simulink model "SMC_POS_SMC_Att"  (R2024b)
settings: Solver=FixedStepDiscrete  StartTime=0.0  StopTime=45  FixedStep=1/250  RelTol=1e-3
values from neighbouring files (symbols this model uses):
  a1 = 3.5524    [Parameter_SMC.m]
  a2 = 10.000    (= 10)    [Parameter_SMC.m]
  a3 = 8.1910    (= 8.191)    [Parameter_SMC.m]
  a4 = 2.7640    (= 2.764)    [Parameter_SMC.m]
  b3 = 0.6373    [Parameter_SMC.m]
  b4 = 0.0223    [Parameter_SMC.m]
  b_1x = 0.7426    [Parameter_SMC.m]
  b_1y = 0.5930    (= 0.593)    [Parameter_SMC.m]
  b_2x = 1.4305    [Parameter_SMC.m]
  b_2y = 1.0895    [Parameter_SMC.m]
  c_x = 0.2871    [Parameter_SMC.m]
  c_y = 0.3867    [Parameter_SMC.m]
  epsilon_1_a = 0.5    [Parameter_SMC.m]
  epsilon_1_b = 0.5    [Parameter_SMC.m]
  epsilon_2 = 0.5    [Parameter_SMC.m]
  epsilon_2_b = 0.5    [Parameter_SMC.m]
  g = 9.81    [Parameter_SMC.m]
  Jx = 0.005    [Parameter_SMC.m]
  Jy = 0.005    [Parameter_SMC.m]
  Jz = 0.009    [Parameter_SMC.m]
  K1 = 0.01    [Parameter_SMC.m]
  k1 = 0.001    [Parameter_SMC.m]
  K2 = 0    [Parameter_SMC.m]
  k2 = a1    (= 3.5524)    [Parameter_SMC.m]
  k3 = 0.1    [Parameter_SMC.m]
  k4 = 0.5000    (= 0.5)    [Parameter_SMC.m]
  k5 = 0.0388    [Parameter_SMC.m]
  k6 = Jx * a3 / (l * sqrt(8) * Tmax)    [Parameter_SMC.m]
  k7 = 0.3147    [Parameter_SMC.m]
  k8 = a4 * Jz / (4 * Qmax)    (= 0.12438)    [Parameter_SMC.m]
  k_ob = 1    [Parameter_SMC.m]
  l = 0.33/2    (= 0.165)    [Parameter_SMC.m]
  m = 0.8    [Parameter_SMC.m]
  PWM_max = 2000    [Parameter_SMC.m]
  PWM_min = 1000    [Parameter_SMC.m]
  Qmax = 0.05    [Parameter_SMC.m]
  Tmax = 4    [Parameter_SMC.m]
undefined symbols (not defined in the file or in its folder): d_1_x, DiscIntNeverNeededParam, k_1_a, k_1_b, k_2_a, k_2_b, K_4, Q_max, T_max
libraries: simulink x13, slpidlib x3
(part 2 of 2)

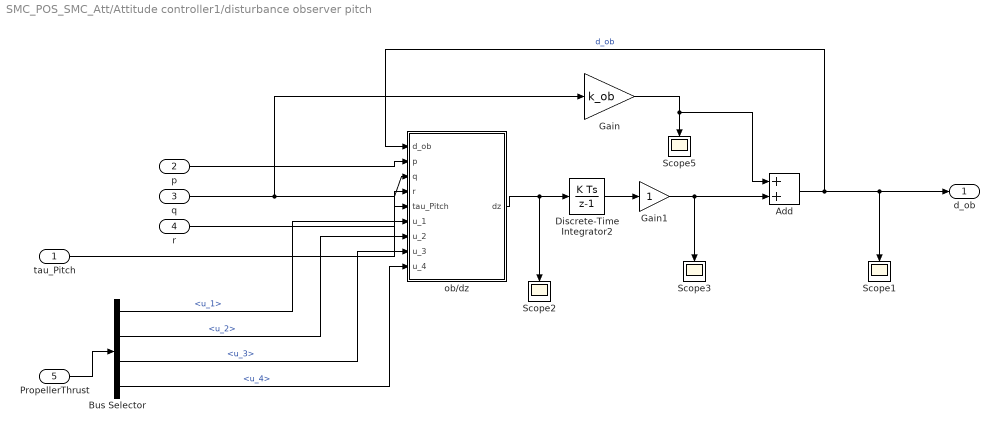
== system SMC_POS_SMC_Att/Attitude controller1/disturbance observer pitch ==
  tau_Pitch : Inport
  "p " : Inport  Port=2
  q : Inport  Port=3
  r : Inport  Port=4
  PropellerThrust : Inport  Port=5
  Add : Sum
  Bus Selector : BusSelector  OutputSignals=u_1,u_2,u_3,u_4
  Discrete-Time Integrator2 : DiscreteIntegrator  SampleTime=-1  ICPrevOutput=DiscIntNeverNeededParam  ICPrevScaledInput=DiscIntNeverNeededParam
  Gain : Gain  Gain=k_ob
  Gain1 : Gain
  Scope{1..3,5} (4 alike) : Scope
  ob/dz : MATLAB Function  TreatAsAtomicUnit=on
  d_ob : Outport
  wires:
  ob/dz/1(dz) -> Discrete-Time Integrator2/1, Scope2/1
  Discrete-Time Integrator2/1 -> Gain1/1
  Gain/1 -> Scope5/1, Add/1
  Add/1 -> Scope1/1, d_ob/1, ob/dz/1(d_ob)  "d_ob"
  Gain1/1 -> Add/2, Scope3/1
  tau_Pitch/1 -> ob/dz/5(tau_Pitch)
  r/1 -> ob/dz/4(r)
  q/1 -> ob/dz/3(q), Gain/1
  "p "/1 -> ob/dz/2(p)
  PropellerThrust/1 -> Bus Selector/1
  Bus Selector/1 -> ob/dz/6(u_1)  "<u_1>"
  Bus Selector/2 -> ob/dz/7(u_2)  "<u_2>"
  Bus Selector/3 -> ob/dz/8(u_3)  "<u_3>"
  Bus Selector/4 -> ob/dz/9(u_4)  "<u_4>"

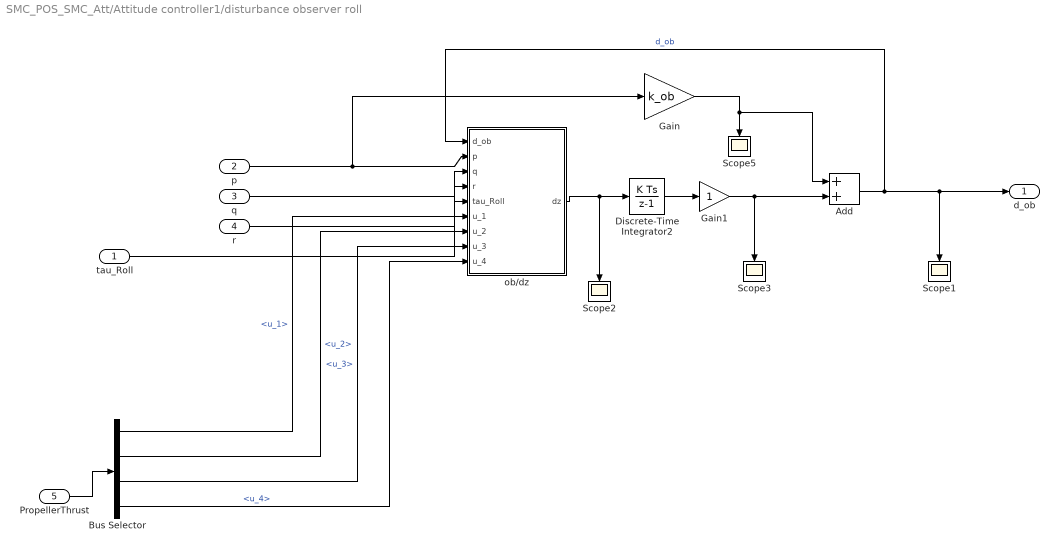
== system SMC_POS_SMC_Att/Attitude controller1/disturbance observer roll ==
  tau_Roll : Inport
  "p " : Inport  Port=2
  q : Inport  Port=3
  r : Inport  Port=4
  PropellerThrust : Inport  Port=5
  Add : Sum
  Bus Selector : BusSelector  OutputSignals=u_1,u_2,u_3,u_4
  Discrete-Time Integrator2 : DiscreteIntegrator  SampleTime=-1  ICPrevOutput=DiscIntNeverNeededParam  ICPrevScaledInput=DiscIntNeverNeededParam
  Gain : Gain  Gain=k_ob
  Gain1 : Gain
  Scope{1..3,5} (4 alike) : Scope
  ob/dz : MATLAB Function  TreatAsAtomicUnit=on
  d_ob : Outport
  wires:
  ob/dz/1(dz) -> Discrete-Time Integrator2/1, Scope2/1
  Discrete-Time Integrator2/1 -> Gain1/1
  Gain/1 -> Scope5/1, Add/1
  Add/1 -> Scope1/1, d_ob/1, ob/dz/1(d_ob)  "d_ob"
  Gain1/1 -> Add/2, Scope3/1
  tau_Roll/1 -> ob/dz/5(tau_Roll)
  r/1 -> ob/dz/4(r)
  q/1 -> ob/dz/3(q)
  "p "/1 -> Gain/1, ob/dz/2(p)
  Bus Selector/4 -> ob/dz/9(u_4)  "<u_4>"
  Bus Selector/3 -> ob/dz/8(u_3)  "<u_3>"
  Bus Selector/1 -> ob/dz/6(u_1)  "<u_1>"
  PropellerThrust/1 -> Bus Selector/1
  Bus Selector/2 -> ob/dz/7(u_2)  "<u_2>"

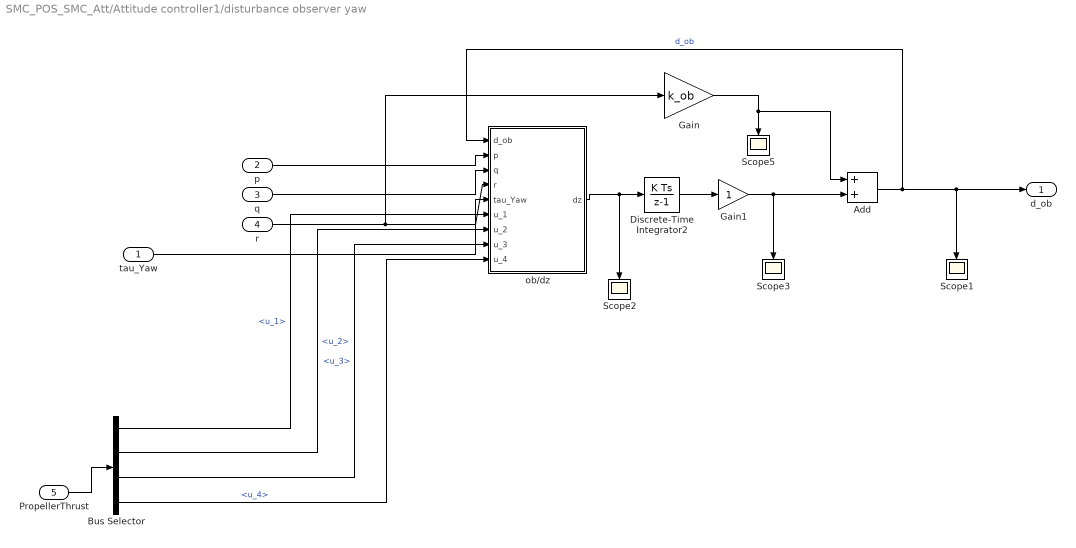
== system SMC_POS_SMC_Att/Attitude controller1/disturbance observer yaw ==
  tau_Yaw : Inport
  "p " : Inport  Port=2
  q : Inport  Port=3
  r : Inport  Port=4
  PropellerThrust : Inport  Port=5
  Add : Sum
  Bus Selector : BusSelector  OutputSignals=u_1,u_2,u_3,u_4
  Discrete-Time Integrator2 : DiscreteIntegrator  SampleTime=-1  ICPrevOutput=DiscIntNeverNeededParam  ICPrevScaledInput=DiscIntNeverNeededParam
  Gain : Gain  Gain=k_ob
  Gain1 : Gain
  Scope{1..3,5} (4 alike) : Scope
  ob/dz : MATLAB Function  TreatAsAtomicUnit=on
  d_ob : Outport
  wires:
  ob/dz/1(dz) -> Discrete-Time Integrator2/1, Scope2/1
  Discrete-Time Integrator2/1 -> Gain1/1
  Gain/1 -> Scope5/1, Add/1
  Add/1 -> Scope1/1, d_ob/1, ob/dz/1(d_ob)  "d_ob"
  Gain1/1 -> Add/2, Scope3/1
  tau_Yaw/1 -> ob/dz/5(tau_Yaw)
  r/1 -> Gain/1, ob/dz/4(r)
  q/1 -> ob/dz/3(q)
  "p "/1 -> ob/dz/2(p)
  Bus Selector/4 -> ob/dz/9(u_4)  "<u_4>"
  Bus Selector/3 -> ob/dz/8(u_3)  "<u_3>"
  Bus Selector/1 -> ob/dz/6(u_1)  "<u_1>"
  PropellerThrust/1 -> Bus Selector/1
  Bus Selector/2 -> ob/dz/7(u_2)  "<u_2>"

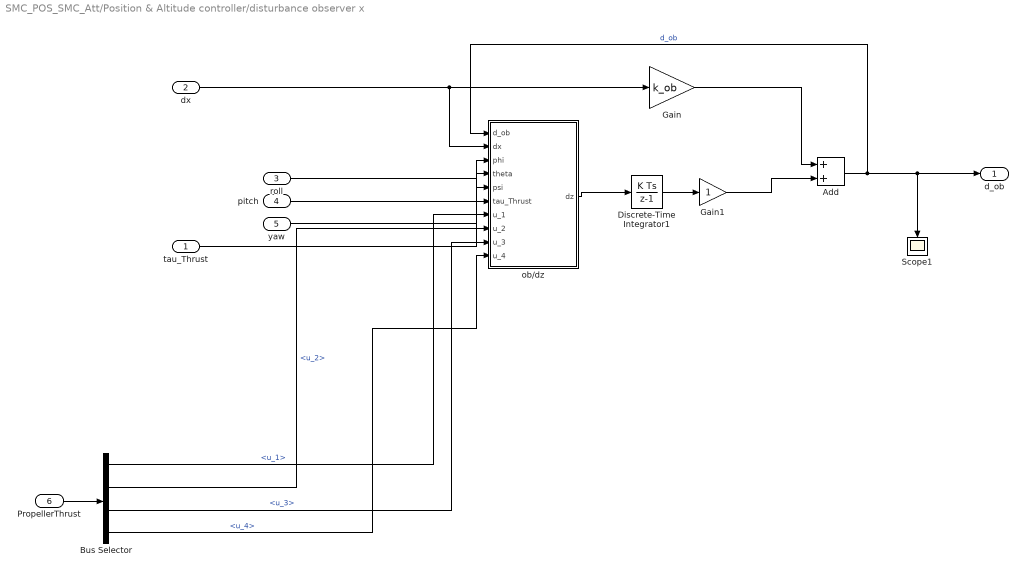
== system SMC_POS_SMC_Att/Position & Altitude controller/disturbance observer x ==
  tau_Thrust : Inport
  dx : Inport  Port=2
  "roll " : Inport  Port=3
  pitch : Inport  Port=4
  yaw : Inport  Port=5
  PropellerThrust : Inport  Port=6
  Add : Sum
  Bus Selector : BusSelector  OutputSignals=u_1,u_2,u_3,u_4
  Discrete-Time Integrator1 : DiscreteIntegrator  SampleTime=-1  ICPrevOutput=DiscIntNeverNeededParam  ICPrevScaledInput=DiscIntNeverNeededParam
  Gain : Gain  Gain=k_ob
  Gain1 : Gain
  Scope1 : Scope
  ob/dz : MATLAB Function  TreatAsAtomicUnit=on
  d_ob : Outport
  wires:
  tau_Thrust/1 -> ob/dz/6(tau_Thrust)
  ob/dz/1(dz) -> Discrete-Time Integrator1/1
  Discrete-Time Integrator1/1 -> Gain1/1
  Gain/1 -> Add/1
  Add/1 -> Scope1/1, d_ob/1, ob/dz/1(d_ob)  "d_ob"
  Gain1/1 -> Add/2
  "roll "/1 -> ob/dz/3(phi)
  pitch/1 -> ob/dz/4(theta)
  yaw/1 -> ob/dz/5(psi)
  dx/1 -> ob/dz/2(dx), Gain/1
  Bus Selector/2 -> ob/dz/8(u_2)  "<u_2>"
  PropellerThrust/1 -> Bus Selector/1
  Bus Selector/4 -> ob/dz/10(u_4)  "<u_4>"
  Bus Selector/1 -> ob/dz/7(u_1)  "<u_1>"
  Bus Selector/3 -> ob/dz/9(u_3)  "<u_3>"

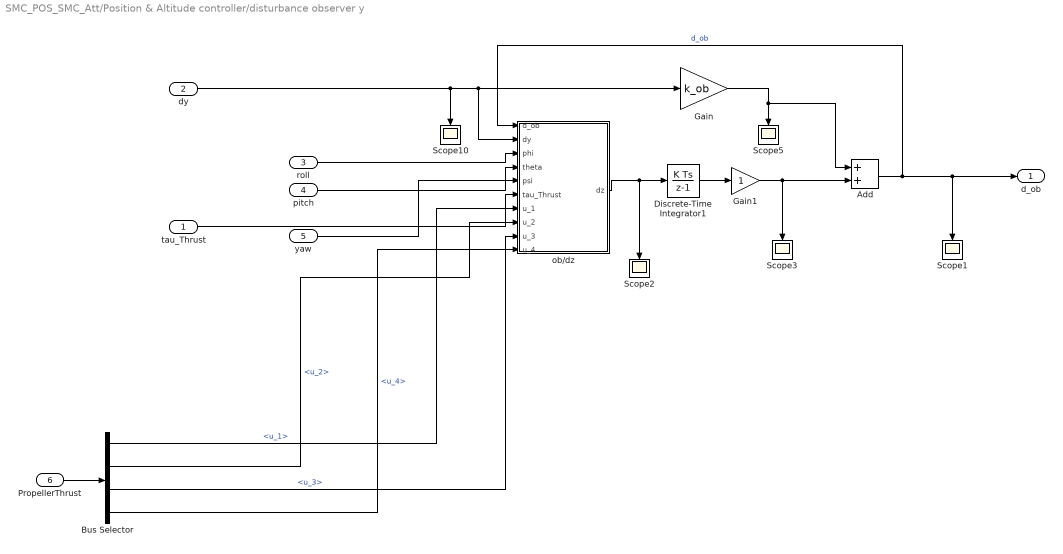
== system SMC_POS_SMC_Att/Position & Altitude controller/disturbance observer y ==
  tau_Thrust : Inport
  dy : Inport  Port=2
  "roll " : Inport  Port=3
  pitch : Inport  Port=4
  yaw : Inport  Port=5
  PropellerThrust : Inport  Port=6
  Add : Sum
  Bus Selector : BusSelector  OutputSignals=u_1,u_2,u_3,u_4
  Discrete-Time Integrator1 : DiscreteIntegrator  SampleTime=-1  ICPrevOutput=DiscIntNeverNeededParam  ICPrevScaledInput=DiscIntNeverNeededParam
  Gain : Gain  Gain=k_ob
  Gain1 : Gain
  Scope{1..3,5,10} (5 alike) : Scope
  ob/dz : MATLAB Function  TreatAsAtomicUnit=on
  d_ob : Outport
  wires:
  tau_Thrust/1 -> ob/dz/6(tau_Thrust)
  ob/dz/1(dz) -> Discrete-Time Integrator1/1, Scope2/1
  Gain/1 -> Scope5/1, Add/1
  Add/1 -> Scope1/1, d_ob/1, ob/dz/1(d_ob)  "d_ob"
  Gain1/1 -> Add/2, Scope3/1
  "roll "/1 -> ob/dz/3(phi)
  pitch/1 -> ob/dz/4(theta)
  yaw/1 -> ob/dz/5(psi)
  dy/1 -> ob/dz/2(dy), Gain/1, Scope10/1
  Discrete-Time Integrator1/1 -> Gain1/1
  Bus Selector/2 -> ob/dz/8(u_2)  "<u_2>"
  PropellerThrust/1 -> Bus Selector/1
  Bus Selector/4 -> ob/dz/10(u_4)  "<u_4>"
  Bus Selector/1 -> ob/dz/7(u_1)  "<u_1>"
  Bus Selector/3 -> ob/dz/9(u_3)  "<u_3>"

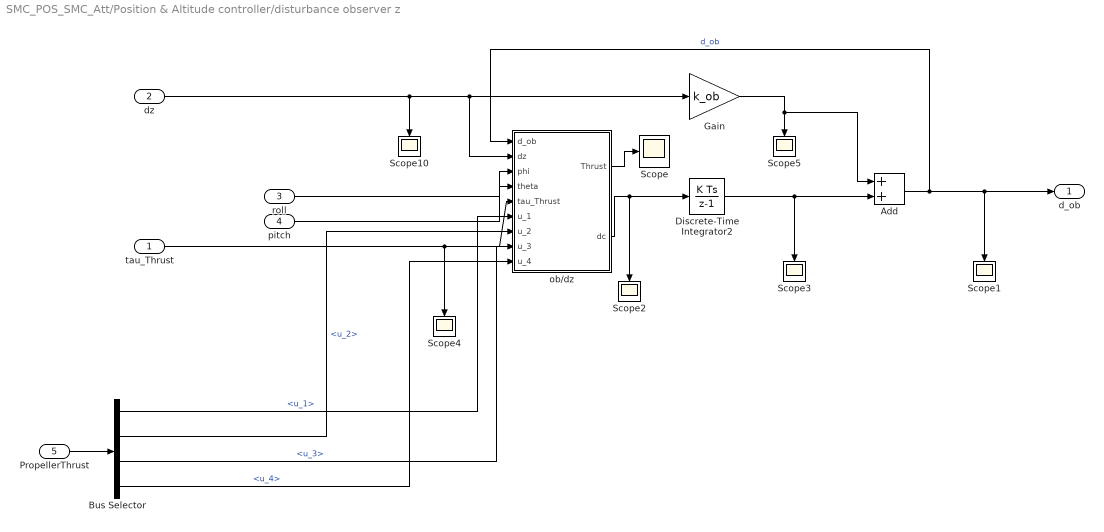
== system SMC_POS_SMC_Att/Position & Altitude controller/disturbance observer z ==
  tau_Thrust : Inport
  dz : Inport  Port=2
  "roll " : Inport  Port=3
  pitch : Inport  Port=4
  PropellerThrust : Inport  Port=5
  Add : Sum
  Bus Selector : BusSelector  OutputSignals=u_1,u_2,u_3,u_4
  Discrete-Time Integrator2 : DiscreteIntegrator  SampleTime=-1  ICPrevOutput=DiscIntNeverNeededParam  ICPrevScaledInput=DiscIntNeverNeededParam
  Gain : Gain  Gain=k_ob
  Scope{,1..5,10} (7 alike) : Scope
  ob/dz : MATLAB Function  TreatAsAtomicUnit=on
  d_ob : Outport
  wires:
  Gain/1 -> Scope5/1, Add/1
  Add/1 -> Scope1/1, d_ob/1, ob/dz/1(d_ob)  "d_ob"
  "roll "/1 -> ob/dz/3(phi)
  pitch/1 -> ob/dz/4(theta)
  tau_Thrust/1 -> Scope4/1, ob/dz/5(tau_Thrust)
  dz/1 -> Gain/1, ob/dz/2(dz), Scope10/1
  ob/dz/2(dc) -> Discrete-Time Integrator2/1, Scope2/1
  Discrete-Time Integrator2/1 -> Add/2, Scope3/1
  ob/dz/1(Thrust) -> Scope/1
  Bus Selector/4 -> ob/dz/9(u_4)  "<u_4>"
  Bus Selector/3 -> ob/dz/8(u_3)  "<u_3>"
  Bus Selector/1 -> ob/dz/6(u_1)  "<u_1>"
  PropellerThrust/1 -> Bus Selector/1
  Bus Selector/2 -> ob/dz/7(u_2)  "<u_2>"

== matlab function SMC_POS_SMC_Att/Position & Altitude controller/Calculate roll and pitch angles  ==
  data: u1 input; theta output; u2 input; psi input; phi output
function [theta,phi] = fcn(u1,u2,psi)
int1=u1*sin(psi)-u2*cos(psi);
if int1 >1 
    int1 =1; 
else if int1 <-1 
        int1=-1;
    else 
        int1=int1;
    end
end
phi=asin(int1);
if phi>1.5 
    phi_2=1.5;
else if phi<-1.5
        phi_2=-1.5;
    else
        phi_2=phi;
    end
end
int2=(u1*cos(psi)+u2*sin(psi))/cos(phi_2);
if int2 >1 
    int2 =1; 
else if int2 <-1 
        int2=-1;
    else 
        int2=int2;
    end
end
theta=asin(int2);
end

== matlab function SMC_POS_SMC_Att/Attitude controller1/MATLAB Function6 ==
  data: roll input; p output; pitch input; yaw input; q output; r output; droll input; dpitch input; dyaw input
function [p, q, r] = fcn(roll,pitch,yaw, droll, dpitch, dyaw)
p=droll-sin(pitch)*dyaw;
q=cos(roll)*dpitch+cos(pitch)*sin(roll)*dyaw;
r=-sin(roll)*dpitch+cos(pitch)*cos(roll)*dyaw;
end

== matlab function SMC_POS_SMC_Att/Position & Altitude controller/Sliding Mode Surface2 ==
  data: error_dz output; sz output; error_z input; dz input; a2 parameter; epsilon_2_b parameter; des_dz input
function [error_dz,sz] = fcn(error_z,dz, a2, epsilon_2_b,des_dz)
error_dz=dz-des_dz;

sz=(a2*error_z+error_dz)/epsilon_2_b;

end

== matlab function SMC_POS_SMC_Att/Position & Altitude controller/Control law3 ==
  data: error_dz input; K1 parameter; k3 parameter; k4 parameter; sgn input; s input; dz input; u output; g parameter; m parameter; phi input; theta input; Tmax parameter; error_z input; b3 parameter; b4 parameter; des_ddz input
 function u  = fcn( error_dz,K1, k3,k4,sgn,s,dz,g, m, phi, theta,Tmax,error_z, b3, b4, des_ddz)
 
 kint=(b3*abs(error_z)+b4*abs(error_dz));
 
 if kint<k3
    kint=k3;
end
if abs(s)<1
u=kint*s+k4/(cos(theta)*cos(phi))*(error_dz)+(-K1*dz*abs(dz)+m*g-m*des_ddz)/(4*Tmax*cos(phi)*cos(theta))+1;
else
%   u=k_3_b*sgn+k_4_b*(error_dz)+(K_3*dz+m*g)/(4*T_max*cos(phi)*cos(theta))+1
    u=kint*sgn+k4/(cos(theta)*cos(phi))*(error_dz)+(-K1*dz*abs(dz)+m*g-m*des_ddz)/(4*Tmax*cos(phi)*cos(theta))+1;
end

== matlab function SMC_POS_SMC_Att/Position & Altitude controller/Sliding Mode Surface ==
  data: sx output; error_x input; error_dx output; error_y input; dx input; dy input; error_dy output; sy output; a1 parameter; epsilon_2 parameter; des_dx input; des_dy input
function [sx,error_dx,error_dy,sy] = fcn(error_x,error_y,dx,dy,a1,epsilon_2,des_dx, des_dy)
error_dx=dx-des_dx;
error_dy=dy-des_dy;
sx=(a1*error_x+error_dx)/epsilon_2;
sy=(a1*error_y+error_dy)/epsilon_2;

end

== matlab function SMC_POS_SMC_Att/Attitude controller1/MATLAB Function ==
  data: error_phi input; dphi input; dtheta input; s_phi output; error_theta input; error_dphi output; s_theta output; error_dtheta output; epsilon_1_a parameter; a3 parameter; des_dphi input; des_dtheta input
function [s_phi,error_dphi,s_theta,error_dtheta] = fcn(error_phi, dphi, dtheta,error_theta,epsilon_1_a, a3, des_dphi, des_dtheta)
error_dphi=dphi-des_dphi;
error_dtheta=dtheta-des_dtheta;

s_phi=(a3*error_phi+error_dphi)/epsilon_1_a;
s_theta=(a3*error_theta+error_dtheta)/epsilon_1_a;

== matlab function SMC_POS_SMC_Att/Attitude controller1/derivative1/MATLAB Function7 ==
  data: u input; y output
function y = fcn(u)
if abs(u)>30 
    u=0;
end
y = u;

== matlab function SMC_POS_SMC_Att/Position & Altitude controller/Control law1 ==
  data: error_x input; d_ob input; dx input; K1 parameter; k1 parameter; k2 parameter; sgn input; s input; error_dx input; g parameter; m parameter; u output; theta input; phi input; b_1x parameter; b_2x parameter; des_ddx input; c_x parameter
 function u = fcn(error_x, d_ob,dx,K1, k1,k2,sgn,s,error_dx,g, m, theta, phi, b_1x, b_2x, des_ddx, c_x)

%      if abs(s)<1
%  u=(k_3*s+k_4*(error_dx)+K_1*dx/(m*g))-d_ob*m*reci_Thrust
% else
%      u=(k_3*sgn+k_4*(error_dx)+K_1*dx/(m*g))-d_ob*m*reci_Thrust
% 
%      end
% (k_3-0.2*(1.5^(-abs(error_x))-1))
%      if abs(s)<1
%  u=(k_3*s+k_4*(error_dx)+K_1*dx/(m*g))-d_ob*m*reci_Thrust
% else
%      u=((k_3-0.2*(1.5^(-abs(error_x))-1))*sgn+k_4*(error_dx)+K_1*dx/(m*g))-d_ob*m*reci_Thrust
% 
%      end
% %   kint=(0.08*abs(error_x)-0.13*abs(error_dx));clear all


  kint=(b_1x*abs(error_x)+b_2x*abs(error_dx));

if kint<k1
    kint=k1;
end
if abs(s)<1
 u=(kint*(cos(phi)*cos(theta)/g)*s+k2*(cos(phi)*cos(theta)/g)*error_dx-K1*(cos(phi)*cos(theta)/(m*g))*dx*abs(dx)-(cos(phi)*cos(theta)/g)*des_ddx+c_x*(cos(phi)*cos(theta)/g)*s)+d_ob*(cos(phi)*cos(theta)/g);
%   u=(kint*s+k_4*cos(theta)*cos(phi)*error_dx+K_1*cos(theta)*cos(phi)*dx/(m*g)-cos(theta)*cos(phi)*des_ddx/g)-d_ob*m*reci_Thrust
else    
% u=((k_3-0.2*(1.5^(-abs(error_x))-1))*sgn+k_4*(error_dx)+K_1*dx/(m*g))-d_ob*m*reci_Thrust
% u=((0.05*abs(error_x)-0.065*abs(error_dx))*sgn+k_4*(error_dx)+K_1*dx/(m*g))-d_ob*m*reci_Thrust
 u=(kint*(cos(phi)*cos(theta)/g)*sgn+k2*(cos(phi)*cos(theta)/g)*error_dx-K1*(cos(phi)*cos(theta)/(m*g))*dx*abs(dx)-(cos(phi)*cos(theta)/g)*des_ddx+c_x*(cos(phi)*cos(theta)/g)*s)+d_ob*(cos(phi)*cos(theta)/g);
%   u=(kint*sgn+k_4*cos(theta)*cos(phi)*error_dx+K_1*cos(theta)*cos(phi)*dx/(m*g)-cos(theta)*cos(phi)*des_ddx/g)-d_ob*m*reci_Thrust
end

== matlab function SMC_POS_SMC_Att/Attitude controller1/derivative3/MATLAB Function7 ==
  data: u input; y output
function y = fcn(u)
if abs(u)>30 
    u=0;
end
y = u;

== matlab function SMC_POS_SMC_Att/Attitude controller1/MATLAB Function3 ==
  data: error input; s_psi output; dpsi input; error_dpsi output; a4 parameter; epsilon_1_b parameter; des_dpsi input
function [s_psi,error_dpsi] = fcn(error,dpsi,a4, epsilon_1_b, des_dpsi)
error_psi=error;
error_dpsi=dpsi-des_dpsi;
s_psi=(a4*error_psi+error_dpsi)/epsilon_1_b;

== matlab function SMC_POS_SMC_Att/Attitude controller1/derivative10/MATLAB Function7 ==
  data: u input; y output
function y = fcn(u)
if abs(u)>30 
    u=0;
end
y = u;

== matlab function SMC_POS_SMC_Att/Position & Altitude controller/disturbance observer x/ob//dz ==
  data: d_ob input; dx input; m parameter; PWM_min parameter; PWM_max parameter; phi input; theta input; psi input; dz output; Tmax parameter; tau_Thrust input; k_ob parameter; K1 parameter; u_1 input; u_2 input; u_3 input; u_4 input
 function  dz = fcn(d_ob, dx, m, PWM_min, PWM_max, phi,theta,psi, Tmax, tau_Thrust, k_ob, K1, u_1, u_2, u_3, u_4)
u_x=sin(phi)*sin(psi)+cos(phi)*sin(theta)*cos(psi);
Thrust = -Tmax*(4000*(tau_Thrust)-4*PWM_min)/(PWM_max-PWM_min);
% dz = -k_ob*d_ob - k_ob*(1/m*u_x*Thrust- (K_1*dx)/m);
% test= k_ob*1/m*u_x*Thrust;
dz = -k_ob*d_ob - k_ob*(1/m*u_x*(-Tmax*(u_1+u_2+u_3+u_4))- (K1*dx*abs(dx))/m);

end

== matlab function SMC_POS_SMC_Att/Position & Altitude controller/disturbance observer y/ob//dz ==
  data: d_ob input; dy input; m parameter; PWM_min parameter; PWM_max parameter; phi input; theta input; psi input; dz output; Tmax parameter; tau_Thrust input; k_ob parameter; K1 parameter; u_1 input; u_2 input; u_3 input; u_4 input
 function dz  = fcn(d_ob, dy, m, PWM_min, PWM_max, phi,theta,psi, Tmax, tau_Thrust, k_ob, K1, u_1, u_2, u_3, u_4)
u_y=-sin(phi)*cos(psi)+cos(phi)*sin(theta)*sin(psi);
Thrust = -Tmax*(4000*(tau_Thrust)-4*PWM_min)/(PWM_max-PWM_min);
% dz = -k_ob*d_ob - k_ob*(1/m*u_y*Thrust- (K_1*dy)/m);
% test= k_ob*1/m*u_x*Thrust;
dz = -k_ob*d_ob - k_ob*(1/m*u_y*(-Tmax*(u_1+u_2+u_3+u_4))- (K1*dy*abs(dy))/m);

end

== matlab function SMC_POS_SMC_Att/Attitude controller1/disturbance observer pitch/ob//dz ==
  data: d_ob input; Tmax parameter; k_ob parameter; K2 parameter; p input; dz output; q input; r input; tau_Pitch input; Jz parameter; Jy parameter; Jx parameter; l parameter; u_1 input; u_2 input; u_3 input; u_4 input
 function dz  = fcn(d_ob,  Tmax,  k_ob, K2, p, q, r, tau_Pitch, Jz, Jy, Jx, l, u_1, u_2, u_3, u_4)

%dz = -k_ob*d_ob - k_ob/Jy*(-T_max*l*sqrt(2)/2*(4*tau_Pitch)-K_2*q-p*r*(Jx-Jz));

dz = -k_ob*d_ob - k_ob/Jy*(-Tmax*(u_2*(l*sqrt(2)/2)+ u_4*(l*sqrt(2)/2)- u_1*(l*sqrt(2)/2)- u_3*(l*sqrt(2)/2))-K2*q*abs(q)-p*r*(Jx-Jz));

end

== matlab function SMC_POS_SMC_Att/Dynamic model /Dynamic model ==
  data: channel input double size=4; ddx output size=1; phi input; theta input; psi input; Qmax parameter; Tmax parameter; g parameter; dx input; dy input; dz input; p input; q input; r input; Jy parameter; Jz parameter; Jx parameter; m parameter; ddy output size=1; ddz output size=1; dp output size=1; dq output size=1; dr output size=1; K1 parameter; K2 parameter; l parameter; PWM_max parameter; PWM_min parameter; d_f_x input; d_f_y input; d_f_z input; d_t_p input; d_t_q input; d_t_r input; bias_x input; bias_y input; u_1 output size=1; u_2 output size=1; u_3 output size=1; u_4 output size=1
 function [ddx,ddy,ddz,dp,dq,dr,u_1,u_2,u_3,u_4] =...
     fcn(channel,phi,theta,psi,Qmax,Tmax,g,dx,dy,dz,p,q,r, Jy, Jz, Jx, m,K1, K2, l, PWM_max, PWM_min, d_f_x, d_f_y, d_f_z, d_t_p, d_t_q, d_t_r, bias_x, bias_y)
 
%propeller speed, dutycycle
for index = 1:4
    if channel(index)<PWM_min
    channel(index)=PWM_min;
            else if channel(index)>PWM_max
             channel(index)=PWM_max;
                else
             channel(index)=channel(index);
                 end
    end
end
%,u_2,u_3,u_4
u_1=(channel(1)-PWM_min)/(PWM_max-PWM_min);
u_2=(channel(2)-PWM_min)/(PWM_max-PWM_min);
u_3=(channel(3)-PWM_min)/(PWM_max-PWM_min);
u_4=(channel(4)-PWM_min)/(PWM_max-PWM_min);

ddx = (sin(phi)*sin(psi)+cos(phi)*sin(theta)*cos(psi))*(-Tmax*(u_1+u_2+u_3+u_4))/m - (K1*dx*abs(dx))/m + d_f_x;
ddy = (-sin(phi)*cos(psi)+cos(phi)*sin(theta)*sin(psi))*(-Tmax*(u_1+u_2+u_3+u_4))/m - (K1*dy*abs(dy))/m + d_f_y;
ddz = g + (cos(phi)*cos(theta))*(-Tmax*(u_1+u_2+u_3+u_4))/m - (K1*dz*abs(dz))/m + d_f_z;

% roll
dp = (-Tmax*(u_1*(l*sqrt(2)/2-bias_y)+ u_4*(l*sqrt(2)/2-bias_y)- u_2*(l*sqrt(2)/2+bias_y)- u_3*(l*sqrt(2)/2+bias_y)) - K2*p*abs(p) - q*r*(Jz-Jy))/Jx + d_t_p;

% pitch
dq = (-Tmax*(u_2*(l*sqrt(2)/2+bias_x)+ u_4*(l*sqrt(2)/2+bias_x)- u_1*(l*sqrt(2)/2-bias_x)- u_3*(l*sqrt(2)/2-bias_x)) - K2*q*abs(q) - p*r*(Jx-Jz))/Jy + d_t_q;

%yaw
dr = (Qmax*(u_1+u_2-u_3-u_4) - K2*r*abs(r) - p*q*(Jy-Jx))/Jz + d_t_r;

== matlab function SMC_POS_SMC_Att/Position & Altitude controller/disturbance observer z/ob//dz ==
  data: Thrust output; d_ob input; dz input; m parameter; PWM_min parameter; PWM_max parameter; phi input; theta input; dc output; Tmax parameter; tau_Thrust input; k_ob parameter; K1 parameter; g parameter; u_1 input; u_2 input; u_3 input; u_4 input
 function  [Thrust, dc] = fcn(d_ob, dz, m, PWM_min, PWM_max, phi,theta, Tmax, tau_Thrust, k_ob, K1,g, u_1, u_2, u_3, u_4)
u_z=cos(phi)*cos(theta);
Thrust = -Tmax*(4000*(tau_Thrust)-4*PWM_min)/(PWM_max-PWM_min);
%dc = -k_ob*d_ob - k_ob*(g+1/m*u_z*Thrust- (K_1*dz)/m);
% test= k_ob*1/m*u_x*Thrust;
% dc = -k_ob*d_ob - k_ob*(g+1/m*u_z*(-T_max*(u_1+u_2+u_3+u_4))- (K_1*dz)/m);
dc = -k_ob*d_ob - k_ob*(g+1/m*u_z*(-Tmax*(u_1+u_2+u_3+u_4))- (K1*dz*abs(dz))/m);
end

== matlab function SMC_POS_SMC_Att/Position & Altitude controller/MATLAB Function ==
  data: tau_Thrust_og input; tau_Thrust output; d_ob input; phi input; theta input; m parameter; Tmax parameter
function tau_Thrust= fcn(tau_Thrust_og, d_ob, phi, theta, m, Tmax)

tau_Thrust = tau_Thrust_og+ d_ob*m/(4*Tmax*cos(theta)*cos(phi)) ;
end

== matlab function SMC_POS_SMC_Att/Dynamic model /Rotation Matrix ==
  data: p input; dphi output; dtheta output; dpsi output; q input; r input; phi input; theta input
function [dphi,dtheta,dpsi] = fcn(p,q,r,phi,theta)

%roll
dphi=p+q*sin(phi)*tan(theta)+r*cos(phi)*tan(theta);

%pitch
dtheta=q*cos(phi)-r*sin(phi);

%yaw
dpsi=q*sin(phi)/cos(theta)+r*cos(phi)/cos(theta);
% dphi=p
% dtheta=q
% dpsi=r

== matlab function SMC_POS_SMC_Att/Attitude controller1/disturbance observer roll/ob//dz ==
  data: d_ob input; Tmax parameter; k_ob parameter; K2 parameter; p input; dz output; q input; r input; tau_Roll input; Jz parameter; Jy parameter; Jx parameter; l parameter; u_1 input; u_2 input; u_3 input; u_4 input
 function dz  = fcn(d_ob,  Tmax,  k_ob, K2, p, q, r, tau_Roll, Jz, Jy, Jx, l, u_1, u_2, u_3, u_4)

% dz = -k_ob*d_ob - k_ob/Jx*(-T_max*l*sqrt(2)/2*(4*tau_Roll)-K_2*p-q*r*(Jz-Jy));
dz = -k_ob*d_ob - k_ob/Jx*(-Tmax*(u_1*(l*sqrt(2)/2)+ u_4*(l*sqrt(2)/2)- u_2*(l*sqrt(2)/2)- u_3*(l*sqrt(2)/2))-K2*p*abs(p)-q*r*(Jz-Jy));
end

== matlab function SMC_POS_SMC_Att/Attitude controller1/disturbance observer yaw/ob//dz ==
  data: d_ob input; Qmax parameter; k_ob parameter; K2 parameter; p input; dz output; q input; r input; tau_Yaw input; Jz parameter; Jy parameter; Jx parameter; u_1 input; u_2 input; u_3 input; u_4 input
 function dz  = fcn(d_ob,  Qmax,  k_ob, K2, p, q, r, tau_Yaw, Jz, Jy, Jx, u_1, u_2, u_3, u_4)

% dz = -k_ob*d_ob - k_ob/Jz*(Q_max*(4*tau_Yaw)-K_2*r-q*p*(Jy-Jx));
dz = -k_ob*d_ob - k_ob/Jz*(Qmax*(u_1+u_2-u_3-u_4)-K2*r*abs(r)-q*p*(Jy-Jx));
end

== matlab function SMC_POS_SMC_Att/Attitude controller1/MATLAB Function5 ==
  data: roll input; p output; pitch input; yaw input; q output; r output; droll input; dpitch input; dyaw input
function [p, q, r] = fcn(roll,pitch,yaw, droll, dpitch, dyaw)
p=droll-sin(pitch)*dyaw;
q=cos(roll)*dpitch+cos(pitch)*sin(roll)*dyaw;
r=-sin(roll)*dpitch+cos(pitch)*cos(roll)*dyaw;
end

== matlab function SMC_POS_SMC_Att/Attitude controller1/MATLAB Function7 ==
  data: s_p input; tau_roll output; s_q input; s_r input; sgn_p input; sgn_q input; sgn_r input; error_p input; error_q input; error_r input; d_ob_p input; d_ob_q input; d_ob_r input; k_1_a parameter; k_2_a parameter; T_max parameter; d_1_x parameter; p input; q input; r input; Jy parameter; tau_pitch output; tau_yaw output; Jx parameter; Jz parameter; K_4 parameter; k_1_b parameter; k_2_b parameter; Q_max parameter
function [tau_roll, tau_pitch, tau_yaw] = fcn( s_p, s_q, s_r,sgn_p, sgn_q, sgn_r, error_p, error_q, error_r,d_ob_p, d_ob_q, d_ob_r, k_1_a, k_2_a, T_max, d_1_x, p, q, r, Jy,Jx, Jz, K_4,k_1_b, k_2_b, Q_max)
if  abs(s_p)< 1
tau_roll= k_1_a*s_p+k_2_a*error_p - (q*r*(Jz-Jy)+K_4*p)/(T_max*d_1_x*4) +d_ob_p*Jx/(T_max*d_1_x*4);
else if abs(s_p)>= 1
tau_roll= k_1_a*sgn_p+k_2_a*error_p - (q*r*(Jz-Jy)+K_4*p)/(T_max*d_1_x*4) +d_ob_p*Jx/(T_max*d_1_x*4);
    end
end

if  abs(s_q)< 1
tau_pitch= k_1_a*s_q+k_2_a*error_q - (p*r*(Jx-Jz)+K_4*q)/(T_max*d_1_x*4) +d_ob_q*Jy/(T_max*d_1_x*4);
else if abs(s_q)>= 1
tau_pitch= k_1_a*sgn_q+k_2_a*error_q - (p*r*(Jx-Jz)+K_4*q)/(T_max*d_1_x*4) +d_ob_q*Jy/(T_max*d_1_x*4);
    end
end

if  abs(s_r)< 1
tau_yaw= -k_1_b*s_r-k_2_b*error_r + (p*q*(Jy-Jx)+K_4*r)/(Q_max*4) -d_ob_r*Jz/(Q_max*4);
else if abs(s_r)>= 1
tau_yaw= -k_1_b*sgn_r-k_2_b*error_r + (p*q*(Jy-Jx)+K_4*r)/(Q_max*4) -d_ob_r*Jz/(Q_max*4);
end
end

== matlab function SMC_POS_SMC_Att/Attitude controller1/MATLAB Function8 ==
  data: s input; sgn input; sat_theta output
function sat_theta = fcn( s, sgn )
if  abs(s)< 1
sat_theta = s;
else
sat_theta = sgn;
end

== matlab function SMC_POS_SMC_Att/Attitude controller1/MATLAB Function9 ==
  data: s input; sgn input; sat_psi output
function sat_psi = fcn( s, sgn )
if  abs(s)< 1
sat_psi = s;
else
sat_psi = sgn;
end

== matlab function SMC_POS_SMC_Att/Attitude controller1/MATLAB Function10 ==
  data: s input; sgn input; sat_phi output
function sat_phi = fcn( s, sgn )
if  abs(s)< 1
sat_phi = s;
else
sat_phi = sgn;
end

== matlab function SMC_POS_SMC_Att/Attitude controller1/MATLAB Function12 ==
  data: tau_pitch output size=1; sat_phi input; sat_theta input; sat_psi input; tau_roll output size=1; error_dphi input; error_dtheta input; error_dpsi input; k5 parameter; k6 parameter; d_ob_phi input; d_ob_theta input; d_ob_psi input; Jx parameter; Tmax parameter; l parameter; tau_yaw output size=1; k7 parameter; k8 parameter; p input; q input; r input; phi input; theta input; dphi input; dtheta input; des_ddphi input; des_ddtheta input; des_ddpsi input; K2 parameter; Qmax parameter; Jy parameter; Jz parameter
function [tau_pitch, tau_roll, tau_yaw] = fcn( sat_phi, sat_theta, sat_psi,error_dphi, error_dtheta, error_dpsi, k5, k6,...
    d_ob_phi, d_ob_theta, d_ob_psi, Jx, Tmax, l, k7, k8, p, q, r, phi, theta, dphi, dtheta, des_ddphi, des_ddtheta, des_ddpsi,K2, Qmax, Jy, Jz)

fa1 = q*((1/cos(theta)^2)*dtheta*sin(phi)+tan(theta)*cos(phi)*dphi)+r*((1/cos(theta)^2)*dtheta*cos(phi)-tan(theta)*sin(phi)*dphi);
fa2 = fa1-((Jz-Jy)/Jx)*q*r-K2*p*abs(p)/Jx-((Jx-Jz)/Jy)*p*r*tan(theta)*sin(phi)-K2*q*abs(q)*tan(theta)*sin(phi)/Jy-((Jy-Jx)/Jz)*p*q*tan(theta)*cos(phi)-K2*r*abs(r)*tan(theta)*cos(phi)/Jz;
fb1 = -(q*sin(phi)*dphi+r*cos(phi)*dphi);
fb2 = fb1-(((Jx-Jz)/Jy)*p*r*cos(phi)+K2*q*abs(q)*cos(phi)/Jy+((Jy-Jx)/Jz)*p*q*sin(phi)+K2*r*abs(r)*sin(phi)/Jz);
fc1 = q*(cos(phi)*dphi*cos(theta)+sin(phi)*sin(theta)*dtheta)/cos(theta)^2+r*(cos(phi)*sin(theta)*dtheta-sin(phi)*dphi*cos(theta))/cos(theta)^2;
fc2 = fc1-cos(phi)*(Jy-Jx)*q*p/(cos(theta)*Jz)-(cos(phi)*K2*r*abs(r))/(cos(theta)*Jz)-(sin(phi)*(Jx-Jz)*p*r)/(cos(theta)*Jy)-(sin(phi)*K2*q*abs(q))/(cos(theta)*Jy);

A = [ 1, Jx*tan(theta)*sin(phi)/Jy, -(Jx*4*Qmax*tan(theta)*cos(phi))/(Jz*2*l*sqrt(2)*Tmax);
    0, 1, (Jy*tan(phi)*4*Qmax)/(Jz*2*l*sqrt(2)*Tmax);
    0, -(Jz*tan(phi)*2*l*sqrt(2)*Tmax)/(Jy*4*Qmax), 1 ];
B = [k5*sat_phi+k6*error_dphi+Jx*(fa2-des_ddphi)/(2*l*sqrt(2)*Tmax);
    k5*sat_theta+(k6/cos(phi))*error_dtheta+Jy*(fb2-des_ddtheta)/(2*l*sqrt(2)*Tmax*cos(phi));
    -k7*sat_psi-k8*(cos(theta)/cos(phi))*error_dpsi-cos(theta)*Jz*(fc2-des_ddpsi)/(4*Qmax*cos(phi))];

ans = linsolve(A,B);

tau_roll = ans(1)+d_ob_phi*Jx/(Tmax*2*l*sqrt(2));
tau_pitch = ans(2)+d_ob_theta*Jy/(Tmax*2*l*sqrt(2));
tau_yaw = ans(3)-d_ob_psi*Jz/(Qmax*4);

== matlab function SMC_POS_SMC_Att/Attitude controller1/MATLAB Function11 ==
  data: s_p input; tau_roll output; s_q input; s_r input; sgn_p input; sgn_q input; sgn_r input; error_p input; error_q input; error_r input; d_ob_p input; d_ob_q input; d_ob_r input; k_1_a parameter; k_2_a parameter; T_max parameter; d_1_x parameter; p input; q input; r input; Jy parameter; tau_pitch output; tau_yaw output; Jx parameter; Jz parameter; K_4 parameter; k_1_b parameter; k_2_b parameter; Q_max parameter
function [tau_roll, tau_pitch, tau_yaw] = fcn( s_p, s_q, s_r,sgn_p, sgn_q, sgn_r, error_p, error_q, error_r,d_ob_p, d_ob_q, d_ob_r, k_1_a, k_2_a, T_max, d_1_x, p, q, r, Jy,Jx, Jz, K_4,k_1_b, k_2_b, Q_max)
if  abs(s_p)< 1
tau_roll= k_1_a*s_p+k_2_a*error_p - (q*r*(Jz-Jy)+K_4*p)/(T_max*d_1_x*4) +d_ob_p*Jx/(T_max*d_1_x*4);
else if abs(s_p)>= 1
tau_roll= k_1_a*sgn_p+k_2_a*error_p - (q*r*(Jz-Jy)+K_4*p)/(T_max*d_1_x*4) +d_ob_p*Jx/(T_max*d_1_x*4);
    end
end

if  abs(s_q)< 1
tau_pitch= k_1_a*s_q+k_2_a*error_q - (p*r*(Jx-Jz)+K_4*q)/(T_max*d_1_x*4) +d_ob_q*Jy/(T_max*d_1_x*4);
else if abs(s_q)>= 1
tau_pitch= k_1_a*sgn_q+k_2_a*error_q - (p*r*(Jx-Jz)+K_4*q)/(T_max*d_1_x*4) +d_ob_q*Jy/(T_max*d_1_x*4);
    end
end

if  abs(s_r)< 1
tau_yaw= -k_1_b*s_r-k_2_b*error_r + (p*q*(Jy-Jx)+K_4*r)/(Q_max*4) -d_ob_r*Jz/(Q_max*4);
else if abs(s_r)>= 1
tau_yaw= -k_1_b*sgn_r-k_2_b*error_r + (p*q*(Jy-Jx)+K_4*r)/(Q_max*4) -d_ob_r*Jz/(Q_max*4);
end
end

== matlab function SMC_POS_SMC_Att/Reference Values/MATLAB Function ==
  data: t input; pos output; vel output; acc output; jerk output; snap output
function [pos, vel, acc, jerk, snap] = ref_traj(t)
%#codegen
% pos: 논문과 동일한 "이상적 스텝" (외부 목표/평가지표 기준)
% vel,acc,jerk,snap: 위 스텝의 "C^4 스무딩 복사본"에서 계산(Controller 5용)

    % ===== 논문 스텝 시각/크기 (Drones 2022, 6, 261, §3.1.1) =====
    x0=0; x1=4;      t0x=15;
    y0=0; y1=4;      t0y=15;
    z0=0; z1=-20;    t0z=5;      % NED(z-down) 가정
    yaw0=0; yaw1=pi/2; t0yaw=40; % 90 deg

    % ===== 전환시간(짧게! 미분 가능화 목적) =====
    Tx=1.1; Ty=1.1; Tz=1.2; Tyaw=0.8;

    % ===== raw step: 외부 목표(Controller 1 포함) / 성능평가 기준 =====
    H = @(tt,t0) double(tt >= t0);
    x_raw   = x0 + (x1 - x0)*H(t,t0x);
    y_raw   = y0 + (y1 - y0)*H(t,t0y);
    z_raw   = z0 + (z1 - z0)*H(t,t0z);
    yaw_raw = wrapToPi(yaw0 + wrapToPi(yaw1 - yaw0)*H(t,t0yaw));
    pos = [x_raw; y_raw; z_raw; yaw_raw];

    % ===== smooth copy(C^4) — Controller 5가 미분만 사용할 값 생성 =====
    [x,dx,ddx,jx,sx]     = quintic_step(t,t0x,Tx,x0,x1);
    [y,dy,ddy,jy,sy]     = quintic_step(t,t0y,Ty,y0,y1);
    [z,dz,ddz,jz,sz]     = quintic_step(t,t0z,Tz,z0,z1);
    [yaw,dyaw,ddyaw,jyaw,syaw] = quintic_yaw(t,t0yaw,Tyaw,yaw0,yaw1);

    % 파생량만 사용 (pos는 raw step 유지가 핵심)
    vel  = [dx; dy; dz; dyaw];
    acc  = [ddx; ddy; ddz; ddyaw];
    jerk = [jx; jy; jz; jyaw];
    snap = [sx; sy; sz; syaw];
end

function [p,v,a,j,sn] = quintic_step(t,t0,T,y0,y1)
% 전환구간 [t0,t0+T]만 5차 S-curve(콤팩트 서포트, C^4)
    if T <= 0
        p = y0 + (y1-y0)*double(t>=t0); v=0; a=0; j=0; sn=0; return
    end
    tau = (t - t0)/T;
    if tau<=0, sig=0; d1=0; d2=0; d3=0; d4=0;
    elseif tau>=1, sig=1; d1=0; d2=0; d3=0; d4=0;
    else
        tt=tau; tt2=tt*tt; tt3=tt2*tt; tt4=tt3*tt;
        sig = 10*tt3 - 15*tt4 + 6*tt4*tt;
        d1  = (30*tt2 - 60*tt3 + 30*tt4)/T;
        d2  = (60*tt - 180*tt2 + 120*tt3)/(T*T);
        d3  = (60 - 360*tt + 360*tt2)/(T*T*T);
        d4  = (-360 + 720*tt)/(T*T*T*T);
    end
    A  = (y1 - y0);
    p  = y0 + A*sig;
    v  = A*d1;
    a  = A*d2;
    j  = A*d3;
    sn = A*d4;
end

function [yaw,dyaw,ddyaw,jyaw,syaw] = quintic_yaw(t,t0,T,yaw0,yaw1)
% 최단호 Δ로 보간(래핑 방지) + 같은 σ,σ',...,σ⁽⁴⁾ 적용
    d = wrapToPi(yaw1 - yaw0);
    [sig,d1,d2,d3,d4] = sigma_quintic(t,t0,T);
    yaw   = wrapToPi(yaw0 + d*sig);
    dyaw  = d*d1;  ddyaw = d*d2;  jyaw = d*d3;  syaw = d*d4;
end

function [sig,d1,d2,d3,d4] = sigma_quintic(t,t0,T)
    if T<=0, sig=double(t>=t0); d1=0; d2=0; d3=0; d4=0; return; end
    tau=(t-t0)/T;
    if tau<=0, sig=0; d1=0; d2=0; d3=0; d4=0; return; end
    if tau>=1, sig=1; d1=0; d2=0; d3=0; d4=0; return; end
    tt=tau; tt2=tt*tt; tt3=tt2*tt; tt4=tt3*tt;
    sig = 10*tt3 - 15*tt4 + 6*tt4*tt;
    d1  = (30*tt2 - 60*tt3 + 30*tt4)/T;
    d2  = (60*tt - 180*tt2 + 120*tt3)/(T*T);
    d3  = (60 - 360*tt + 360*tt2)/(T*T*T);
    d4  = (-360 + 720*tt)/(T*T*T*T);
end

function y = wrapToPi(u)
    y = mod(u + pi, 2*pi) - pi;
end

== matlab function SMC_POS_SMC_Att/Attitude controller1/derivative2/MATLAB Function7 ==
  data: u input; y output
function y = fcn(u)
if abs(u)>30 
    u=0;
end
y = u;

== matlab function SMC_POS_SMC_Att/Attitude controller1/derivative4/MATLAB Function7 ==
  data: u input; y output
function y = fcn(u)
if abs(u)>30 
    u=0;
end
y = u;

== matlab function SMC_POS_SMC_Att/Attitude controller1/derivative5/MATLAB Function7 ==
  data: u input; y output
function y = fcn(u)
if abs(u)>8 
    u=0;
end
y = u;

== matlab function SMC_POS_SMC_Att/Attitude controller1/derivative6/MATLAB Function7 ==
  data: u input; y output
function y = fcn(u)
if abs(u)>30 
    u=0;
end
y = u;

== matlab function SMC_POS_SMC_Att/Attitude controller1/derivative7/MATLAB Function7 ==
  data: u input; y output
function y = fcn(u)
if abs(u)>30 
    u=0;
end
y = u;

== matlab function SMC_POS_SMC_Att/Attitude controller1/derivative8/MATLAB Function7 ==
  data: u input; y output
function y = fcn(u)
if abs(u)>30 
    u=0;
end
y = u;

== matlab function SMC_POS_SMC_Att/Attitude controller1/derivative9/MATLAB Function7 ==
  data: u input; y output
function y = fcn(u)
if abs(u)>30 
    u=0;
end
y = u;

== matlab function SMC_POS_SMC_Att/Reference Values/MATLAB Function1 ==
  data: pos input; body_rate output; vel input; acc input; jerk input; snap input; body_acc output; euler output; euler_rate output; euler_acc output
function [body_rate, body_acc, euler, euler_rate, euler_acc] = diff_flat (pos, vel, acc, jerk, snap)

    g = 9.80665;
    m = 0.8;
    
    x = pos (1);
    y = pos (2);
    z = pos (3);
    psi = pos (4);

    dx = vel (1);
    dy = vel (2);
    dz = vel (3);
    d_psi = vel (4);

    ddx = acc (1);
    ddy = acc (2);
    ddz = acc (3);
    dd_psi = acc (4);
       
    j_x = jerk (1);
    j_y = jerk (2);
    j_z = jerk (3);
    psi3 = jerk (4);

    snap_x = snap (1);
    snap_y = snap (2);
    snap_z = snap (3);
    psi4 = snap (4);


    s_x = sin (x);
    c_x = cos (x);
    s_y = sin (y);
    c_y = cos (y);
    s_psi = sin (psi);
    c_psi = cos (psi);

    ddx2 = ddx ^2;
    ddy2 = ddy ^2;
    ddz2 = (ddz + g) ^2;

    term = (s_psi * ddx) - (c_psi * ddy);
    term2 = term ^2;
    
    secterm = (s_psi * ddy) + (c_psi * ddx);

    nu = sqrt ((ddx2 + ddy2 + ddz2) * (ddz2 + term2));

    eta = sqrt (ddz2 + term2);

    kappa = sqrt (ddx2 + ddy2 + ddz2);

        % === add guards ===
    eps1  = 1e-8;
    eta   = max(eta, eps1);
    kappa = max(kappa, eps1);
    nu    = max(nu,  eps1);

    w_R_b = zeros (3, 3);

    w_R_b (1, 1) = ((c_psi * ddz2) - (term * ddy)) / nu;
    w_R_b (1, 2) = -(s_psi * (ddz + g)) / eta;
    w_R_b (1, 3) = ddx / kappa;

    w_R_b (2, 1) = ((s_psi * ddz2) + (term * ddx)) / nu;
    w_R_b (2, 2) = (c_psi * (ddz + g)) / eta;
    w_R_b (2, 3) = ddy / kappa;
    
    w_R_b (3, 1) = - ((ddz + g) * secterm) / nu;
    w_R_b (3, 2) = term / eta;
    w_R_b (3, 3) = (ddz + g) / kappa;

    theta = atan2 (secterm, eta);
    phi = atan2 (term, ddz + g);

    s_phi = sin (phi);
    c_phi = cos (phi);
    s_theta = sin (theta);
    c_theta = cos (theta);

    u1 = m * sqrt (ddx2 + ddy2 + ddz2);

    p = (-m / u1) * ((w_R_b (1, 2) * j_x) + (w_R_b (2, 2) * j_y) + (w_R_b (3, 2) * j_z));
    q = (m / u1) * ((w_R_b (1, 1) * j_x) + (w_R_b (2, 1) * j_y) + (w_R_b (3, 1) * j_z));
   
    d_phi = (p + (c_phi * s_theta * d_psi)) / c_theta;
    d_theta = q - (s_phi * d_psi);

    c_theta = max(c_theta, 1e-6);   % d_phi 분모
    u1    = max(m * kappa, 1e-8);   % thrust magnitude

    r = (s_theta * d_phi) + (c_phi * c_theta * d_psi);    

    front = m / u1;
    one = ((w_R_b (1, 2) * snap_x) + (w_R_b (2, 2) * snap_y) + (w_R_b (3, 2) * snap_z));
    two = 2 * ((ddx * j_x) + (ddy * j_y) + ((ddz + g) * j_z)) / kappa;
    d_p = -(front * (one + (p * two))) + (r * q);
    three = ((w_R_b (1, 1) * snap_x) + (w_R_b (2, 1) * snap_y) + (w_R_b (3, 1) * snap_z));
    d_q = (front * (three - (q * two))) - (r * p);

    a_ready = zeros (3, 3);
    a_ready (1, 1) = c_psi;
    a_ready (2, 1) = s_psi;
    a_ready (1, 2) = -(s_psi * (ddz + g)) / eta;
    a_ready (2, 2) = (c_psi * (ddz + g)) / eta;
    a_ready (3, 2) = term / eta;
    a_ready (3, 3) = 1;

    w_R_b_transpose = w_R_b';
    A_s = w_R_b_transpose * a_ready;

    vector_multiply_to_RT = [-d_psi * s_psi; d_psi * c_psi; 0];
    vector_r_p = [-r; 0; p];
    B_s = (w_R_b_transpose * vector_multiply_to_RT) * d_phi + (vector_r_p * d_theta);

    ph1 = A_s (2, 2) * (d_p - B_s (1));
    ph2 = A_s (1, 2) * (B_s (2) - d_q);
    ph3 = (A_s (1, 2) * A_s (2, 3)) - (A_s (1, 3) * A_s (2, 2));
    ph4 = dd_psi * ph3;

    th1 = A_s (2, 1) * (d_p - B_s (1));
    th2 = A_s (1, 1) * (B_s (2) - d_q);
    th3 = (A_s (1, 1) * A_s (2, 3)) - (A_s (1, 3) * A_s (2, 1));
    th4 = dd_psi * th3;

    den = (A_s (2, 2) * A_s (1, 1)) - (A_s (1, 2) * A_s (2, 1));
    num_ddphi = ph1 + ph2 + ph4;
    num_ddtheta = th4 - th1 - th2;
    dd_phi = num_ddphi / den;
    dd_theta = num_ddtheta / den;

    d_r = B_s (3) + (A_s (3, 1) * dd_phi) + (A_s (3, 2) * dd_theta) + (A_s (3, 3) * dd_psi);

    body_rate = [-p; -q; r];
    body_acc = [-d_p; -d_q; d_r];
    euler = [-phi; -theta; -psi];
    euler_rate = [-d_phi; -d_theta; d_psi];
    euler_acc = [-dd_phi; -dd_theta; dd_psi];
    
end

== matlab function SMC_POS_SMC_Att/Reference Values/MATLAB Function3 ==
  data: t input; pos output; vel output; acc output; jerk output; snap output
function [pos, vel, acc, jerk, snap] = ref_traj(t)
%#codegen

    pos  = ref_pos(t);
    vel  = ref_vel(t);
    acc  = ref_acc(t);
    jerk = ref_jerk(t);
    snap = ref_snap(t);
end

== matlab function SMC_POS_SMC_Att/MATLAB Function14 ==
  data: dob_switch input; y output; u1 input; u2 input
function y = fcn(dob_switch,u1,u2)
y=0;
if dob_switch == 1
    y = u1;
elseif dob_switch ==0
    y=u2;
 
end

== matlab function SMC_POS_SMC_Att/MATLAB Function3 ==
  data: dob_switch input; y output; u1 input; u2 input
function y = fcn(dob_switch,u1,u2)
y=0;
if dob_switch == 1
    y = u1;
elseif dob_switch ==0
    y=u2;
 
end

== matlab function SMC_POS_SMC_Att/MATLAB Function4 ==
  data: dob_switch input; y output; u1 input; u2 input
function y = fcn(dob_switch,u1,u2)
y=0;
if dob_switch == 1
    y = u1;
elseif dob_switch ==0
    y=u2;
 
end

== matlab function SMC_POS_SMC_Att/MATLAB Function5 ==
  data: dob_switch input; y output; u1 input; u2 input
function y = fcn(dob_switch,u1,u2)
y=0;
if dob_switch == 1
    y = u1;
elseif dob_switch ==0
    y=u2;
 
end

== matlab function SMC_POS_SMC_Att/MATLAB Function6 ==
  data: dob_switch input; y output; u1 input; u2 input
function y = fcn(dob_switch,u1,u2)
y=0;
if dob_switch == 1
    y = u1;
elseif dob_switch ==0
    y=u2;
 
end

== matlab function SMC_POS_SMC_Att/MATLAB Function7 ==
  data: dob_switch input; y output; u1 input; u2 input
function y = fcn(dob_switch,u1,u2)
y=0;
if dob_switch == 1
    y = u1;
elseif dob_switch ==0
    y=u2;
 
end

== matlab function SMC_POS_SMC_Att/Position & Altitude controller/Control law2 ==
  data: error_y input; d_ob input; error_dy input; K1 parameter; k1 parameter; k2 parameter; sgn input; s input; dy input; u output; g parameter; m parameter; kint output; theta input; phi input; b_1y parameter; b_2y parameter; des_ddy input; c_y parameter
 function [u, kint]   = fcn(error_y,d_ob, error_dy,K1, k1,k2,sgn,s,dy,g, m , theta, phi, b_1y, b_2y, des_ddy, c_y) 
% if abs(s)<1
% u=(k_3*s+k_4*(error_dy)+K_2*dy/(m*g))-d_ob*m*reci_Thrust
% else
%     u=(k_3*sgn+k_4*(error_dy)+K_2*dy/(m*g))-d_ob*m*reci_Thrust
% end

% (k_3-0.2*(1.5^(-abs(s))-1))
% (k_3-0.2*(1.5^(-abs(error_y))-1))
% % kint=(0.08*abs(error_y)-0.13*abs(error_dy));

kint=(b_1y*abs(error_y)+b_2y*abs(error_dy));

if kint<k1
    kint=k1;
end
if abs(s)<1
u=(kint*(cos(phi)*cos(theta)/g)*s+k2*(cos(phi)*cos(theta)/g)*error_dy-K1*(cos(phi)*cos(theta)/(m*g))*dy*abs(dy)-(cos(phi)*cos(theta)/g)*des_ddy+c_y*(cos(phi)*cos(theta)/g)*s)+d_ob*(cos(phi)*cos(theta)/g);
else  
% u=((k_3-0.2*(1.5^(-abs(error_y))-1))*sgn+k_4*(error_dy)+K_2*dy/(m*g))-d_ob*m*reci_Thrust
%   u=((0.02*abs(error_y)-0.02*abs(error_dy))*sgn+k_4*(error_dy)+K_2*dy/(m*g))-d_ob*m*reci_Thrust
u=(kint*(cos(phi)*cos(theta)/g)*sgn+k2*(cos(phi)*cos(theta)/g)*error_dy-K1*(cos(phi)*cos(theta)/(m*g))*dy*abs(dy)-(cos(phi)*cos(theta)/g)*des_ddy+c_y*(cos(phi)*cos(theta)/g)*s)+d_ob*(cos(phi)*cos(theta)/g);
end
